simulink model "untit"  (R2015b)
settings: Solver=VariableStepAuto  StartTime=0.0  StopTime=10.0  RelTol=1e-3
libraries: fuzblock x1
settings Model: Creator=陈圣鑫  LastModifiedBy=陈圣鑫

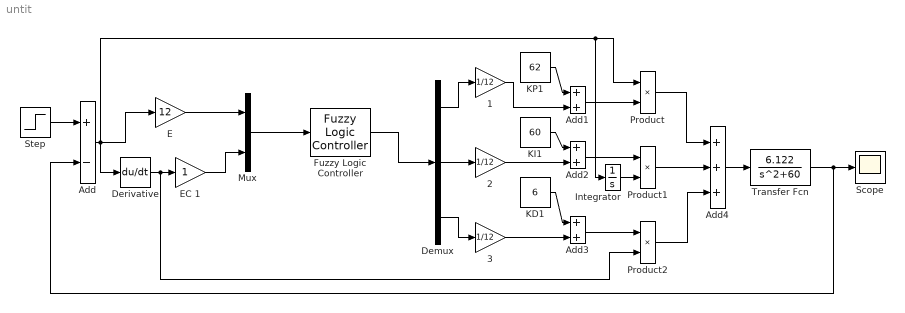
== system untit ==
  "1 " : Gain  Gain=1/12
  "2 " : Gain  Gain=1/12
  3 : Gain  Gain=1/12
  Add : Sum  Inputs=+-
  Add1 : Sum
  Add2 : Sum
  Add3 : Sum
  Add4 : Sum  Inputs=+++
  Demux : Demux  Outputs=3
  Derivative : Derivative
  "E " : Gain  Gain=12
  EC 1 : Gain
  Fuzzy Logic Controller : fuzblock/Fuzzy Logic  Controller  fis=gg
  Integrator : Integrator
  KD1 : Constant  Value=6
  KI1 : Constant  Value=60
  KP1 : Constant  Value=62
  Mux : Mux  Inputs=2
  Product : Product
  Product1 : Product
  Product2 : Product
  Scope : Scope
  Step : Step  SampleTime=0
  Transfer Fcn : TransferFcn  Numerator=[6.122]  Denominator=[1 0 60]
  wires:
  Step/1 -> Add/1
  "E "/1 -> Mux/1
  Add/1 -> Integrator/1, Product/1, Derivative/1, "E "/1
  Derivative/1 -> Product2/2, EC 1/1
  EC 1/1 -> Mux/2
  Mux/1 -> Fuzzy Logic Controller/1
  Fuzzy Logic Controller/1 -> Demux/1
  Demux/1 -> "1 "/1
  Demux/2 -> "2 "/1
  Demux/3 -> 3/1
  "1 "/1 -> Add1/2
  "2 "/1 -> Add2/2
  3/1 -> Add3/2
  KP1/1 -> Add1/1
  KI1/1 -> Add2/1
  KD1/1 -> Add3/1
  Add1/1 -> Product/2
  Add2/1 -> Product1/1
  Add3/1 -> Product2/1
  Product1/1 -> Add4/2
  Product/1 -> Add4/1
  Product2/1 -> Add4/3
  Add4/1 -> Transfer Fcn/1
  Transfer Fcn/1 -> Add/2, Scope/1
  Integrator/1 -> Product1/2
